simulink model "b747_lateral_washout"  (R2025b)
settings: Solver=VariableStepAuto  StartTime=0.0  StopTime=T_end  RelTol=1e-3
undefined symbols (not defined in the file): A, B, C, D, den_wo, K_wo, num_wo, T_end, tau_wo
libraries: simulink_extras x12
settings Model: Creator=임현우  LastModifiedBy=임현우
settings DataIOCC: ReturnWorkspaceOutputsName=out_wo

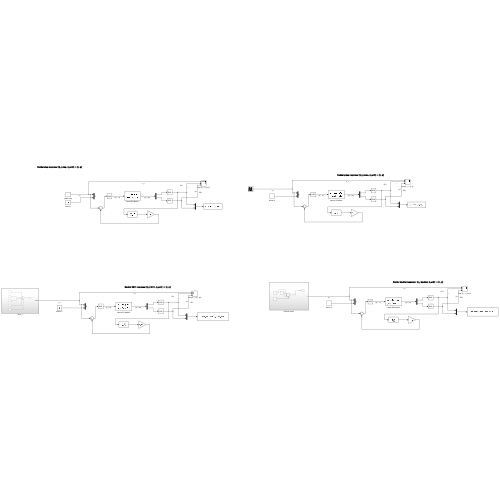
[thumbnail: Simulink's stored preview of the top-level diagram]
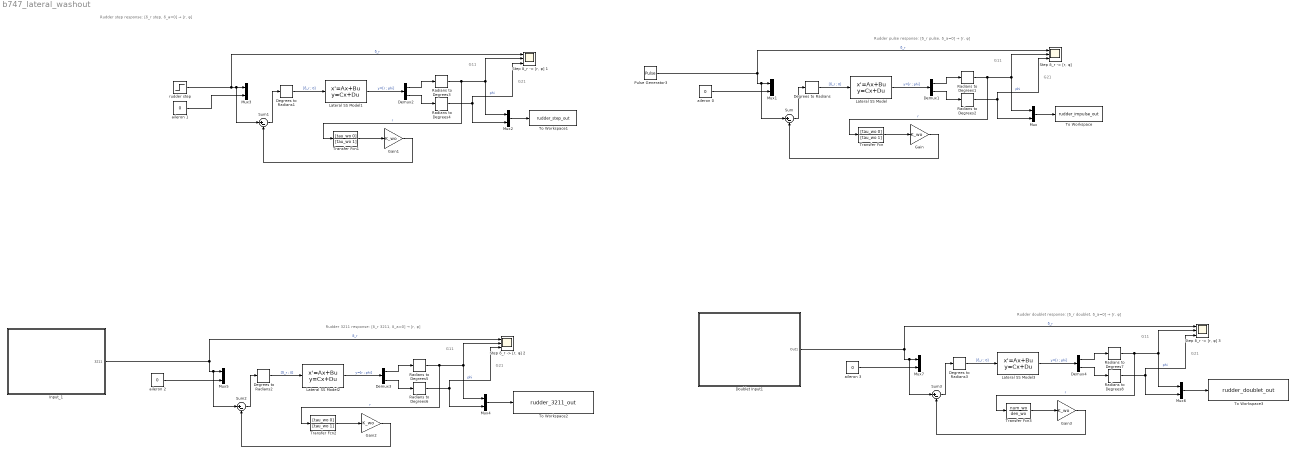
== system b747_lateral_washout ==
  note: Rudder pulse response: [δ_r pulse, δ_a=0] → [r, φ]
  note: G21
  note: G11
  note: G21
  note: Rudder step response: [δ_r step, δ_a=0] → [r, φ]
  note: G11
  note: G11
  note: G21
  note: Rudder 3211 response: [δ_r 3211, δ_a=0] → [r, φ]
  note: Rudder doublet response: [δ_r doublet, δ_a=0] → [r, φ]
  note: G21
  note: G11
  Degrees to Radians{,1..3} (4 alike) : simulink_extras/Transformations/Degrees to Radians
  Demux{1..4} (4 alike) : Demux  Outputs=2
  Doublet Input1 : Subsystem
  Gain{,1..3} (4 alike) : Gain  Gain=K_wo
  Input_1 : Subsystem
  Lateral SS Model{,1..3} (4 alike) : StateSpace  A=A  B=B  C=C  D=D  InitialCondition=0
  Mux{,1..7} (8 alike) : Mux  Inputs=2
  Pulse Generator3 : DiscretePulseGenerator  PulseType=Time based  Amplitude=20  Period=T_end  PulseWidth=0.125  PhaseDelay=1
  Radians to Degrees{1..8} (8 alike) : simulink_extras/Transformations/Radians to Degrees
  Step δ_r -> [r, φ] {,1..3} (4 alike) : Scope  NumInputPorts=3
      "Step δ_r -> [r, φ] " settings: ActiveDisplayYMinimum=-3.0186664292068337  ActiveDisplayYMaximum=4.6952173136128117
      "Step δ_r -> [r, φ] 1" settings: ActiveDisplayYMinimum=-3.0186664292068337  ActiveDisplayYMaximum=4.6952173136128117
      "Step δ_r -> [r, φ] 2" settings: ActiveDisplayYMinimum=-1.5182618860711328  ActiveDisplayYMaximum=2.377773585560194  DataLoggingVariableName=ScopeData2
      "Step δ_r -> [r, φ] 3" settings: ActiveDisplayYMinimum=-1.8333166789737974  ActiveDisplayYMaximum=1.1436219395933456  DataLoggingVariableName=ScopeData3
  Sum{,1..3} (4 alike) : Sum  Inputs=|+-
  To Workspace : ToWorkspace  VariableName=rudder_impulse_out  SaveFormat=Timeseries  SampleTime=-1
  To Workspace1 : ToWorkspace  VariableName=rudder_step_out  SaveFormat=Timeseries  SampleTime=-1
  To Workspace2 : ToWorkspace  VariableName=rudder_3211_out  SaveFormat=Timeseries  SampleTime=-1
  To Workspace3 : ToWorkspace  VariableName=rudder_doublet_out  SaveFormat=Timeseries  SampleTime=-1
  Transfer Fcn : TransferFcn  Numerator=[tau_wo 0]  Denominator=[tau_wo 1]
  Transfer Fcn1 : TransferFcn  Numerator=[tau_wo 0]  Denominator=[tau_wo 1]
  Transfer Fcn2 : TransferFcn  Numerator=[tau_wo 0]  Denominator=[tau_wo 1]
  Transfer Fcn3 : TransferFcn  Numerator=num_wo  Denominator=den_wo
  aileron {0..3} (4 alike) : Constant  Value=0
  rudder step : Step  SampleTime=0
  wires:
  Degrees to Radians/1 -> Lateral SS Model/1  "[δ_r ; 0]"
  Demux1/2 -> Radians to Degrees2/1
  Radians to Degrees1/1 -> Transfer Fcn/1, Mux/1, "Step δ_r -> [r, φ] "/2  "r"
  aileron 0/1 -> Mux1/2
  Demux1/1 -> Radians to Degrees1/1
  Pulse Generator3/1 -> Sum/1, Mux1/1, "Step δ_r -> [r, φ] "/1  "δ_r"
  Lateral SS Model/1 -> Demux1/1  "y=[r ; phi]"
  Radians to Degrees2/1 -> Mux/2, "Step δ_r -> [r, φ] "/3  "phi"
  Transfer Fcn/1 -> Gain/1
  Gain/1 -> Sum/2
  Sum/1 -> Degrees to Radians/1
  Mux/1 -> To Workspace/1
  Mux2/1 -> To Workspace1/1
  rudder step/1 -> "Step δ_r -> [r, φ] 1"/1, Sum1/1, Mux3/1  "δ_r"
  Radians to Degrees4/1 -> Mux2/2, "Step δ_r -> [r, φ] 1"/3  "phi"
  Demux2/1 -> Radians to Degrees3/1
  Demux2/2 -> Radians to Degrees4/1
  Sum1/1 -> Degrees to Radians1/1
  Degrees to Radians1/1 -> Lateral SS Model1/1  "[δ_r ; 0]"
  Radians to Degrees3/1 -> Transfer Fcn1/1, Mux2/1, "Step δ_r -> [r, φ] 1"/2  "r"
  aileron 1/1 -> Mux3/2
  Lateral SS Model1/1 -> Demux2/1  "y=[r ; phi]"
  Transfer Fcn1/1 -> Gain1/1
  Gain1/1 -> Sum1/2
  Mux4/1 -> To Workspace2/1
  Radians to Degrees6/1 -> Mux4/2, "Step δ_r -> [r, φ] 2"/3  "phi"
  Demux3/1 -> Radians to Degrees5/1
  Demux3/2 -> Radians to Degrees6/1
  Sum2/1 -> Degrees to Radians2/1
  Gain2/1 -> Sum2/2
  Transfer Fcn2/1 -> Gain2/1
  Lateral SS Model2/1 -> Demux3/1  "y=[r ; phi]"
  aileron 2/1 -> Mux5/2
  Radians to Degrees5/1 -> Transfer Fcn2/1, Mux4/1, "Step δ_r -> [r, φ] 2"/2  "r"
  Input_1/1(3211) -> Sum2/1, Mux5/1, "Step δ_r -> [r, φ] 2"/1  "δ_r"
  Degrees to Radians2/1 -> Lateral SS Model2/1  "[δ_r ; 0]"
  Doublet Input1/1(Out1) -> Sum3/1, Mux7/1, "Step δ_r -> [r, φ] 3"/1  "δ_r"
  Sum3/1 -> Degrees to Radians3/1
  Mux6/1 -> To Workspace3/1
  Demux4/2 -> Radians to Degrees8/1
  Radians to Degrees8/1 -> Mux6/2, "Step δ_r -> [r, φ] 3"/3  "phi"
  Demux4/1 -> Radians to Degrees7/1
  Degrees to Radians3/1 -> Lateral SS Model3/1  "[δ_r ; 0]"
  aileron 3/1 -> Mux7/2
  Transfer Fcn3/1 -> Gain3/1
  Radians to Degrees7/1 -> Transfer Fcn3/1, Mux6/1, "Step δ_r -> [r, φ] 3"/2  "r"
  Gain3/1 -> Sum3/2
  Lateral SS Model3/1 -> Demux4/1  "y=[r ; phi]"

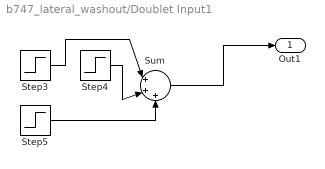
== system b747_lateral_washout/Doublet Input1 ==
  Step3 : Step  Time=2  After=-2  SampleTime=0
  Step4 : Step  SampleTime=0
  Step5 : Step  Time=3  SampleTime=0
  Sum : Sum  Inputs=|+++
  Out1 : Outport
  wires:
  Step4/1 -> Sum/2
  Step5/1 -> Sum/3
  Step3/1 -> Sum/1
  Sum/1 -> Out1/1

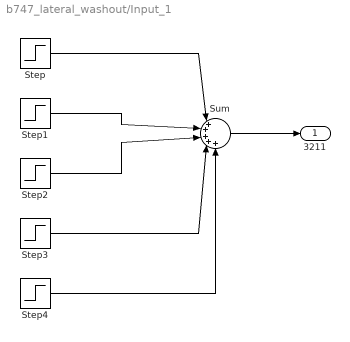
== system b747_lateral_washout/Input_1 ==
  Step : Step  SampleTime=0
  Step1 : Step  Time=4  After=-2  SampleTime=0
  Step2 : Step  Time=6  After=2  SampleTime=0
  Step3 : Step  Time=7  After=-2  SampleTime=0
  Step4 : Step  Time=8  SampleTime=0
  Sum : Sum  Inputs=|+++++
  3211 : Outport
  wires:
  Step/1 -> Sum/1
  Step1/1 -> Sum/2
  Step2/1 -> Sum/3
  Step3/1 -> Sum/4
  Sum/1 -> 3211/1
  Step4/1 -> Sum/5
